simulink model "PSA_mod1"  (R2014a)
settings: Solver=ode45  StartTime=0.0  StopTime=2  RelTol=1e-3
settings Model: Creator=Zero  LastModifiedBy=Zero

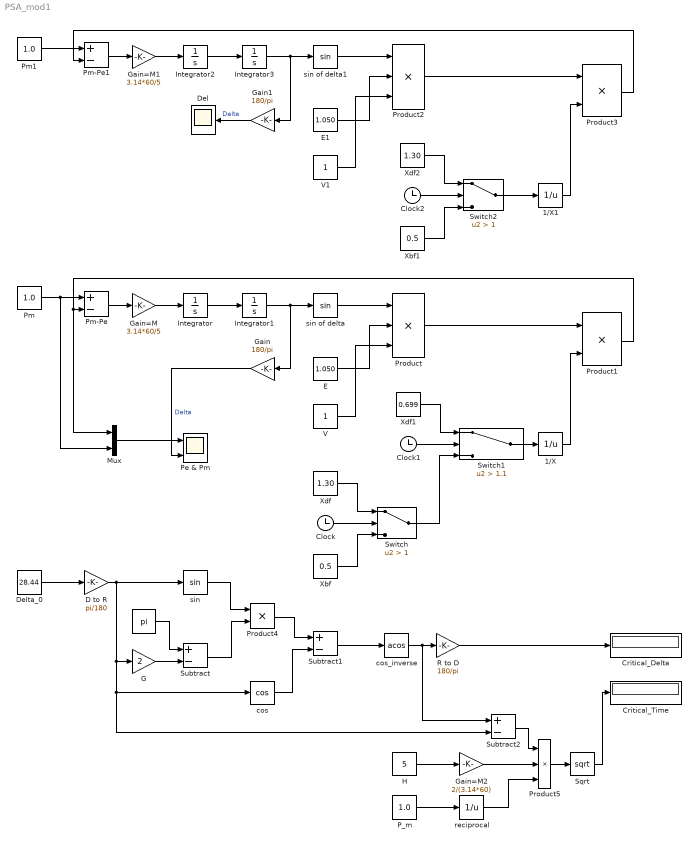
== system PSA_mod1 ==
  " " : Constant  Value=pi
  1/X : Math  Operator=reciprocal  SaturateOnIntegerOverflow=on
  1/X1 : Math  Operator=reciprocal  SaturateOnIntegerOverflow=on
  Clock : Clock
  Clock1 : Clock
  Clock2 : Clock
  Critical_Delta : Display
  Critical_Time : Display
  D to R : Gain  Gain=pi/180
  Del : Scope
  Delta_0 : Constant  Value=28.44
  E : Constant  Value=1.050
  E1 : Constant  Value=1.050
  "G " : Gain  Gain=2
  Gain : Gain  Gain=180/pi
  Gain1 : Gain  Gain=180/pi
  Gain=M : Gain  Gain=3.14*60/5
  Gain=M1 : Gain  Gain=3.14*60/5
  Gain=M2 : Gain  Gain=2/(3.14*60)
  H : Constant  Value=5
  Integrator{,1..3} (4 alike) : Integrator
  Mux : Mux  Inputs=2
  P_m : Constant  Value=1.0
  Pe & Pm : Scope  NumInputPorts=2
      settings: YMin=-5~-5  YMax=5~20
  Pm : Constant  Value=1.0
  Pm-Pe : Sum  Inputs=+-
  Pm-Pe1 : Sum  Inputs=+-
  Pm1 : Constant  Value=1.0
  Product : Product  Inputs=3
  Product1 : Product
  Product2 : Product  Inputs=3
  Product3 : Product
  Product4 : Product
  Product5 : Product  Inputs=3
  R to D : Gain  Gain=180/pi
  Sqrt : Sqrt  SaturateOnIntegerOverflow=on
  Subtract : Sum  Inputs=+-
  Subtract1 : Sum  Inputs=+-
  Subtract2 : Sum  Inputs=+-
  Switch : Switch  Criteria=u2 > Threshold  Threshold=1
  Switch1 : Switch  Criteria=u2 > Threshold  Threshold=1.1
  Switch2 : Switch  Criteria=u2 > Threshold  Threshold=1
  V : Constant
  V1 : Constant
  Xbf : Constant  Value=0.5
  Xbf1 : Constant  Value=0.5
  Xdf : Constant  Value=1.30
  Xdf1 : Constant  Value=0.699
  Xdf2 : Constant  Value=1.30
  cos : Trigonometry  Operator=cos
  cos_inverse : Trigonometry  Operator=acos
  reciprocal : Math  Operator=reciprocal  SaturateOnIntegerOverflow=on
  "sin " : Trigonometry
  sin of delta : Trigonometry
  sin of delta1 : Trigonometry
  wires:
  Pm-Pe/1 -> Gain=M/1
  Gain=M/1 -> Integrator/1
  Integrator/1 -> Integrator1/1
  E/1 -> Product/2
  V/1 -> Product/3
  Product/1 -> Product1/1
  1/X/1 -> Product1/2
  Clock/1 -> Switch/2
  Integrator1/1 -> Gain/1, sin of delta/1
  Mux/1 -> Pe & Pm/1
  Xdf/1 -> Switch/1
  Xbf/1 -> Switch/3
  Gain/1 -> Pe & Pm/2  "Delta"
  Pm/1 -> Mux/2, Pm-Pe/1
  Product1/1 -> Mux/1, Pm-Pe/2
  Clock1/1 -> Switch1/2
  Xdf1/1 -> Switch1/1
  Switch1/1 -> 1/X/1
  Switch/1 -> Switch1/3
  Pm-Pe1/1 -> Gain=M1/1
  Gain=M1/1 -> Integrator2/1
  Integrator2/1 -> Integrator3/1
  sin of delta1/1 -> Product2/1
  E1/1 -> Product2/2
  V1/1 -> Product2/3
  Product2/1 -> Product3/1
  1/X1/1 -> Product3/2
  Clock2/1 -> Switch2/2
  Integrator3/1 -> Gain1/1, sin of delta1/1
  Xdf2/1 -> Switch2/1
  Xbf1/1 -> Switch2/3
  Pm1/1 -> Pm-Pe1/1
  Product3/1 -> Pm-Pe1/2
  Switch2/1 -> 1/X1/1
  Gain1/1 -> Del/1  "Delta"
  Delta_0/1 -> D to R/1
  "sin "/1 -> Product4/1
  Subtract/1 -> Product4/2
  D to R/1 -> Subtract2/2, cos/1, "G "/1, "sin "/1
  "G "/1 -> Subtract/2
  " "/1 -> Subtract/1
  Product4/1 -> Subtract1/1
  cos/1 -> Subtract1/2
  Subtract1/1 -> cos_inverse/1
  cos_inverse/1 -> Subtract2/1, R to D/1
  R to D/1 -> Critical_Delta/1
  Subtract2/1 -> Product5/1
  H/1 -> Gain=M2/1
  Gain=M2/1 -> Product5/2
  P_m/1 -> reciprocal/1
  reciprocal/1 -> Product5/3
  Product5/1 -> Sqrt/1
  Sqrt/1 -> Critical_Time/1
  sin of delta/1 -> Product/1
